simulink model "controllo_con_azione_integrale"  (R2022b)
settings: Solver=VariableStepAuto  StartTime=0.0  StopTime=40  RelTol=1e-3
values from neighbouring files (symbols this model uses):
  Kd_ci = 120    [controllo_script.m]
  Ki_ci = 1e4    (= 10000)    [controllo_script.m]
  Kp_ci = 2100    [controllo_script.m]
  T = T_A * T_B    [DH_dinamica.m]    (also in traiettoria_script.m = 0.001)
  theta1_0 = pi/2 - angolo    [CLIK_script.m]
  theta2_0 = 2*angolo    [CLIK_script.m]
undefined symbols (not defined in the file or in its folder): DiscIntNeverNeededParam
settings Model: Creator=Principale  LastModifiedBy=Michele
settings DataIOCC: ReturnWorkspaceOutputs=off

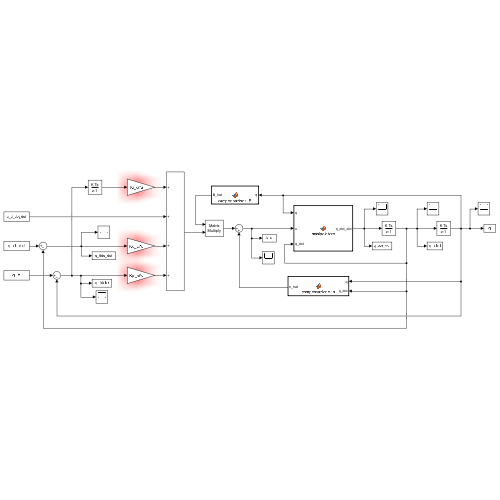
[thumbnail: Simulink's stored preview of the top-level diagram]
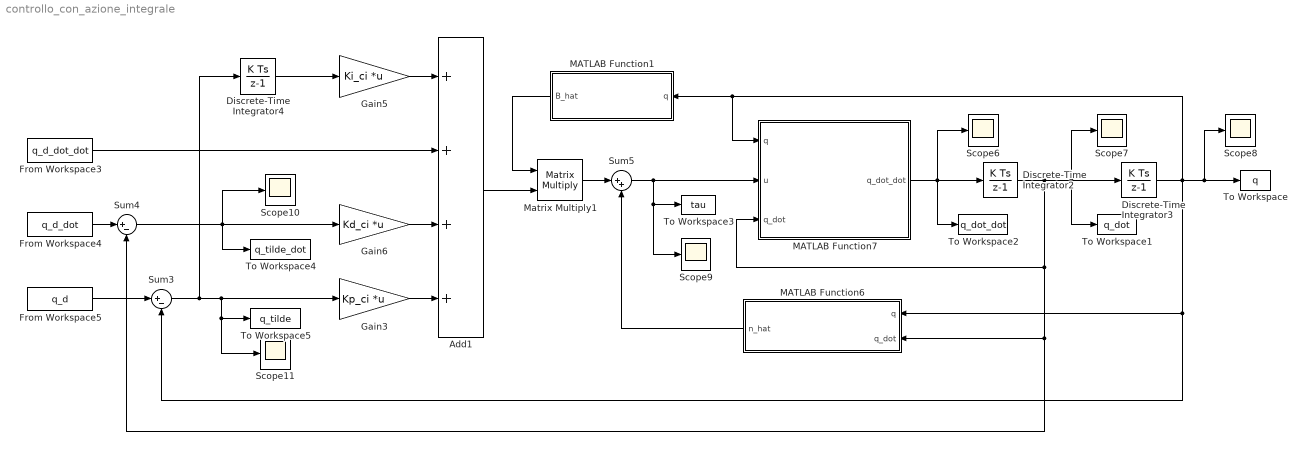
== system controllo_con_azione_integrale ==
  Add1 : Sum  Inputs=++++
  Discrete-Time Integrator2 : DiscreteIntegrator  InitialCondition=[0 0 0 0]'  SampleTime=-1  ICPrevOutput=DiscIntNeverNeededParam  ICPrevScaledInput=DiscIntNeverNeededParam
  Discrete-Time Integrator3 : DiscreteIntegrator  InitialCondition=[theta1_0 theta2_0 -0.25 0]'  SampleTime=-1  ICPrevOutput=DiscIntNeverNeededParam  ICPrevScaledInput=DiscIntNeverNeededParam
  Discrete-Time Integrator4 : DiscreteIntegrator  InitialCondition=[0 0 0 0]'  SampleTime=-1  ICPrevOutput=DiscIntNeverNeededParam  ICPrevScaledInput=DiscIntNeverNeededParam
  From Workspace3 : FromWorkspace  VariableName=q_d_dot_dot  SampleTime=T
  From Workspace4 : FromWorkspace  VariableName=q_d_dot  SampleTime=T
  From Workspace5 : FromWorkspace  VariableName=q_d  SampleTime=T
  Gain3 : Gain  Gain=Kp_ci  Multiplication=Matrix(K*u)
  Gain5 : Gain  Gain=Ki_ci  Multiplication=Matrix(K*u)
  Gain6 : Gain  Gain=Kd_ci  Multiplication=Matrix(K*u)
  MATLAB Function1 : MATLAB Function  TreatAsAtomicUnit=on
  MATLAB Function6 : MATLAB Function  TreatAsAtomicUnit=on
  MATLAB Function7 : MATLAB Function  TreatAsAtomicUnit=on
  Matrix Multiply1 : Product  Multiplication=Matrix(*)
  Scope{6..11} (6 alike) : Scope
  Sum3 : Sum  Inputs=|+-
  Sum4 : Sum  Inputs=|+-
  Sum5 : Sum  Inputs=|++
  To Workspace : ToWorkspace  VariableName=q  SaveFormat=Structure With Time  SampleTime=-1
  To Workspace1 : ToWorkspace  VariableName=q_dot  SaveFormat=Structure With Time  SampleTime=-1
  To Workspace2 : ToWorkspace  VariableName=q_dot_dot  SaveFormat=Structure With Time  SampleTime=-1
  To Workspace3 : ToWorkspace  VariableName=tau  SaveFormat=Structure With Time  SampleTime=-1
  To Workspace4 : ToWorkspace  VariableName=q_tilde_dot  SaveFormat=Structure With Time  SampleTime=-1
  To Workspace5 : ToWorkspace  VariableName=q_tilde  SaveFormat=Structure With Time  SampleTime=-1
  wires:
  From Workspace5/1 -> Sum3/1
  Sum3/1 -> Discrete-Time Integrator4/1, Gain3/1, To Workspace5/1, Scope11/1
  Sum4/1 -> Gain6/1, To Workspace4/1, Scope10/1
  Matrix Multiply1/1 -> Sum5/1
  MATLAB Function1/1(B_hat) -> Matrix Multiply1/1
  Gain5/1 -> Add1/1
  Discrete-Time Integrator2/1 -> Discrete-Time Integrator3/1, To Workspace1/1, Scope7/1, Sum4/2, MATLAB Function6/2(q_dot), MATLAB Function7/3(q_dot)
  MATLAB Function7/1(q_dot_dot) -> Discrete-Time Integrator2/1, Scope6/1, To Workspace2/1
  From Workspace3/1 -> Add1/2
  Gain3/1 -> Add1/4
  From Workspace4/1 -> Sum4/1
  Gain6/1 -> Add1/3
  Add1/1 -> Matrix Multiply1/2
  Sum5/1 -> MATLAB Function7/2(u), Scope9/1, To Workspace3/1
  MATLAB Function6/1(n_hat) -> Sum5/2
  Discrete-Time Integrator3/1 -> To Workspace/1, Scope8/1, Sum3/2, MATLAB Function6/1(q), MATLAB Function7/1(q), MATLAB Function1/1(q)
  Discrete-Time Integrator4/1 -> Gain5/1

== matlab function controllo_con_azione_integrale/MATLAB Function1 ==
  data: q input; B_hat output
function B_hat = compensazione_B(q)

    q1 = q(1);
    q2 = q(2);
    
    B = [10*(cos(q1)/2 + (cos(q1)*cos(q2))/2 - (sin(q1)*sin(q2))/2)^2 + 20*(cos(q1)/2 + (cos(q1)*cos(q2))/4 - (sin(q1)*sin(q2))/4)^2 + 10*(sin(q1)/2 + (cos(q1)*sin(q2))/2 + (cos(q2)*sin(q1))/2)^2 + 20*(sin(q1)/2 + (cos(q1)*sin(q2))/4 + (cos(q2)*sin(q1))/4)^2 + (5*cos(q1)^2)/4 + (5*sin(q1)^2)/4 + 4513/500, 10*((cos(q1)*cos(q2))/2 - (sin(q1)*sin(q2))/2)*(cos(q1)/2 + (cos(q1)*cos(q2))/2 - (sin(q1)*sin(q2))/2) + 20*((cos(q1)*cos(q2))/4 - (sin(q1)*sin(q2))/4)*(cos(q1)/2 + (cos(q1)*cos(q2))/4 - (sin(q1)*sin(q2))/4) + 10*((cos(q1)*sin(q2))/2 + (cos(q2)*sin(q1))/2)*(sin(q1)/2 + (cos(q1)*sin(q2))/2 + (cos(q2)*sin(q1))/2) + 20*((cos(q1)*sin(q2))/4 + (cos(q2)*sin(q1))/4)*(sin(q1)/2 + (cos(q1)*sin(q2))/4 + (cos(q2)*sin(q1))/4) + 627/125, 1/3, -51/50;
    10*((cos(q1)*cos(q2))/2 - (sin(q1)*sin(q2))/2)*(cos(q1)/2 + (cos(q1)*cos(q2))/2 - (sin(q1)*sin(q2))/2) + 20*((cos(q1)*cos(q2))/4 - (sin(q1)*sin(q2))/4)*(cos(q1)/2 + (cos(q1)*cos(q2))/4 - (sin(q1)*sin(q2))/4) + 10*((cos(q1)*sin(q2))/2 + (cos(q2)*sin(q1))/2)*(sin(q1)/2 + (cos(q1)*sin(q2))/2 + (cos(q2)*sin(q1))/2) + 20*((cos(q1)*sin(q2))/4 + (cos(q2)*sin(q1))/4)*(sin(q1)/2 + (cos(q1)*sin(q2))/4 + (cos(q2)*sin(q1))/4) + 627/125, 10*((cos(q1)*cos(q2))/2 - (sin(q1)*sin(q2))/2)^2 + 10*((cos(q1)*sin(q2))/2 + (cos(q2)*sin(q1))/2)^2 + 20*((cos(q1)*cos(q2))/4 - (sin(q1)*sin(q2))/4)^2 + 20*((cos(q1)*sin(q2))/4 + (cos(q2)*sin(q1))/4)^2 + 627/125, 1/4, -51/50;
    1/4, 1/4, 45/2, 0;
    -51/50, -51/50, 0, 7/5];
    
    % Costruisco B_hat estraendo solo i termini sulla diagonale di B
    B_hat = diag(diag(B));   
end

== matlab function controllo_con_azione_integrale/MATLAB Function6 ==
  data: q input; n_hat output; q_dot input
function n_hat = compensazione_n(q,q_dot)

    % n_hat compensa solo la coppia di gravità
    n_hat=[0;0;98.1;0];
end

== matlab function controllo_con_azione_integrale/MATLAB Function7 ==
  data: q input; q_dot_dot output; u input; q_dot input
function q_dot_dot = manipolatore(q, u, q_dot)

    q1 = q(1);
    q2 = q(2);
    q3 = q(3);
    q4 = q(4);
    
    q_dot1 = q_dot(1);
    q_dot2 = q_dot(2);
    q_dot3 = q_dot(3);
    q_dot4 = q_dot(4);
    
    B = [14*(cos(q1)/2 + (cos(q1)*cos(q2))/2 - (sin(q1)*sin(q2))/2)^2 + 20*(cos(q1)/2 + (cos(q1)*cos(q2))/4 - (sin(q1)*sin(q2))/4)^2 + 14*(sin(q1)/2 + (cos(q1)*sin(q2))/2 + (cos(q2)*sin(q1))/2)^2 + 20*(sin(q1)/2 + (cos(q1)*sin(q2))/4 + (cos(q2)*sin(q1))/4)^2 + (5*cos(q1)^2)/4 + (5*sin(q1)^2)/4 + 4513/500, 14*((cos(q1)*cos(q2))/2 - (sin(q1)*sin(q2))/2)*(cos(q1)/2 + (cos(q1)*cos(q2))/2 - (sin(q1)*sin(q2))/2) + 20*((cos(q1)*cos(q2))/4 - (sin(q1)*sin(q2))/4)*(cos(q1)/2 + (cos(q1)*cos(q2))/4 - (sin(q1)*sin(q2))/4) + 14*((cos(q1)*sin(q2))/2 + (cos(q2)*sin(q1))/2)*(sin(q1)/2 + (cos(q1)*sin(q2))/2 + (cos(q2)*sin(q1))/2) + 20*((cos(q1)*sin(q2))/4 + (cos(q2)*sin(q1))/4)*(sin(q1)/2 + (cos(q1)*sin(q2))/4 + (cos(q2)*sin(q1))/4) + 627/125,  1/4, -51/50;
    14*((cos(q1)*cos(q2))/2 - (sin(q1)*sin(q2))/2)*(cos(q1)/2 + (cos(q1)*cos(q2))/2 - (sin(q1)*sin(q2))/2) + 20*((cos(q1)*cos(q2))/4 - (sin(q1)*sin(q2))/4)*(cos(q1)/2 + (cos(q1)*cos(q2))/4 - (sin(q1)*sin(q2))/4) + 14*((cos(q1)*sin(q2))/2 + (cos(q2)*sin(q1))/2)*(sin(q1)/2 + (cos(q1)*sin(q2))/2 + (cos(q2)*sin(q1))/2) + 20*((cos(q1)*sin(q2))/4 + (cos(q2)*sin(q1))/4)*(sin(q1)/2 + (cos(q1)*sin(q2))/4 + (cos(q2)*sin(q1))/4) + 627/125,                                                                                                                                                                                                                         14*((cos(q1)*cos(q2))/2 - (sin(q1)*sin(q2))/2)^2 + 14*((cos(q1)*sin(q2))/2 + (cos(q2)*sin(q1))/2)^2 + 20*((cos(q1)*cos(q2))/4 - (sin(q1)*sin(q2))/4)^2 + 20*((cos(q1)*sin(q2))/4 + (cos(q2)*sin(q1))/4)^2 + 627/125,  1/4, -51/50;
                                                                                                                                                                                                                                                                                                                                                                                                                                           1/4,                                                                                                                                                                                                                                                                                                                                                                                                                                         1/4, 53/2,      0;
                                                                                                                                                                                                                                                                                                                                                                                                                                        -51/50,                                                                                                                                                                                                                                                                                                                                                                                                                                      -51/50,    0,    7/5];
    
    n = [q_dot2/20000 + (q_dot1*(q_dot2*(14*((cos(q1)*sin(q2))/2 + (cos(q2)*sin(q1))/2)*(cos(q1)/2 + (cos(q1)*cos(q2))/2 - (sin(q1)*sin(q2))/2) + 20*((cos(q1)*sin(q2))/4 + (cos(q2)*sin(q1))/4)*(cos(q1)/2 + (cos(q1)*cos(q2))/4 - (sin(q1)*sin(q2))/4) - 14*((cos(q1)*cos(q2))/2 - (sin(q1)*sin(q2))/2)*(sin(q1)/2 + (cos(q1)*sin(q2))/2 + (cos(q2)*sin(q1))/2) - 20*((cos(q1)*cos(q2))/4 - (sin(q1)*sin(q2))/4)*(sin(q1)/2 + (cos(q1)*sin(q2))/4 + (cos(q2)*sin(q1))/4)) + q_dot1*(28*((cos(q1)*sin(q2))/2 + (cos(q2)*sin(q1))/2)*(cos(q1)/2 + (cos(q1)*cos(q2))/2 - (sin(q1)*sin(q2))/2) + 40*((cos(q1)*sin(q2))/4 + (cos(q2)*sin(q1))/4)*(cos(q1)/2 + (cos(q1)*cos(q2))/4 - (sin(q1)*sin(q2))/4) - 28*((cos(q1)*cos(q2))/2 - (sin(q1)*sin(q2))/2)*(sin(q1)/2 + (cos(q1)*sin(q2))/2 + (cos(q2)*sin(q1))/2) - 40*((cos(q1)*cos(q2))/4 - (sin(q1)*sin(q2))/4)*(sin(q1)/2 + (cos(q1)*sin(q2))/4 + (cos(q2)*sin(q1))/4))))/2 - (q_dot1*q_dot2*(14*((cos(q1)*sin(q2))/2 + (cos(q2)*sin(q1))/2)*(cos(q1)/2 + (cos(q1)*cos(q2))/2 - (sin(q1)*sin(q2))/2) + 20*((cos(q1)*sin(q2))/4 + (cos(q2)*sin(q1))/4)*(cos(q1)/2 + (cos(q1)*cos(q2))/4 - (sin(q1)*sin(q2))/4) - 14*((cos(q1)*cos(q2))/2 - (sin(q1)*sin(q2))/2)*(sin(q1)/2 + (cos(q1)*sin(q2))/2 + (cos(q2)*sin(q1))/2) - 20*((cos(q1)*cos(q2))/4 - (sin(q1)*sin(q2))/4)*(sin(q1)/2 + (cos(q1)*sin(q2))/4 + (cos(q2)*sin(q1))/4)))/2];
    
    q_dot_dot = B\(u-n);
end
